simulink model "bb01_quick_start"  (Simulink 7.7)
settings: Solver=FixedStepDiscrete  StartTime=0.0  StopTime=inf  FixedStep=0.002  RelTol=1e-3
PostLoadFcn:
  | qc_set_target_type(getConfigSet(bdroot, 'QUARC Default Target Configuration'));
undefined symbols (not defined in the file): HIL, qc_get_step_size
libraries: quarc_library x5, simulink x2
settings Model: Creator=Rchan  LastModifiedBy=MLevis  SimulationMode=external  ExtModeTrigDuration=5000
settings SolverCC: PositivePriorityOrder=on
settings OptimizationCC: InitFltsAndDblsToZero=on
settings DebuggingCC: SaveWithParameterizedLinksMsg=none  MultiTaskDSMMsg=warning  MultiTaskCondExecSysMsg=none  StrictBusMsg=None
settings RTWCC: SystemTargetFile=quarc_win64.tlc  TemplateMakefile=quarc_default_tmf  Description=QUARC Win64 Target  ProcessScript=quarc_win64_make_rtw_hook
settings STFCustomTargetCC: TargetPreCompLibLocation=C:\PROGRA~3\QUARC\lib\2011a\win64\release  FunctionExecutionProfile=off  GeneratePreprocessorConditionals=Disable all  SystemTargetFile=quarc_win64.tlc
settings GRTTargetCC: TargetPreCompLibLocation=C:\PROGRA~3\QUARC\lib\2011a\win64\release  ParMdlRefBuildCompliant=off  CompOptLevelCompliant=off  MatFileLogging=off  ExtMode=on  ExtModeMexFile=quarc_comm

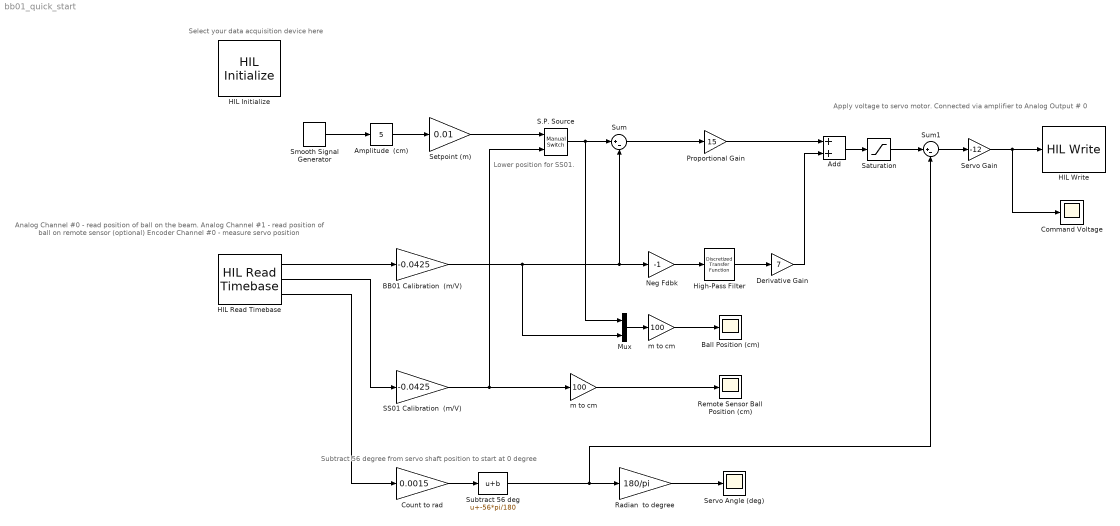
== system bb01_quick_start ==
  note: Select your data acquisition device here
  note: Lower position for SS01.
  note: Analog Channel #0 - read position of ball on the beam.
      | Analog Channel  #1 - read position of ball on remote sensor (optional)
      | Encoder Channel #0 - measure servo position
  note: Apply voltage to servo motor.
      | Connected via amplifier to Analog Output # 0
  note: Subtract 56 degree from servo shaft
      | position to start at 0 degree
  Add : Sum
  Amplitude  (cm) : simulink/Math Operations/Slider Gain  SystemSampleTime=-1  low=-10  gain=5  high=10
  BB01 Calibration  (m/V) : Gain  Gain=-0.0425  SaturateOnIntegerOverflow=on  OutDataTypeStr=Inherit: Same as input  ParamDataTypeStr=Inherit: Same as input
  Ball Position (cm) : Scope
      settings: YMin=-10  YMax=10  SaveName=ScopeData2
  Command Voltage : Scope
      settings: YMin=-10  YMax=10  SaveName=ScopeData3
  Count to rad : Gain  Gain=0.0015  SaturateOnIntegerOverflow=on  OutDataTypeStr=Inherit: Same as input  ParamDataTypeStr=Inherit: Same as input
  Derivative Gain : Gain  Gain=7
  HIL Initialize : quarc_library/Data Acquisition/Generic/Configuration/HIL Initialize  Priority=-99  object_name=HIL-1  board_type=q4  board_number=0  exclusive=off  active=off  hardware_clocks=[0:1]  clock_modes=[0 0]  initial_clock_frequencies=[]  set_clock_params_at_start=on  set_clock_params_at_switch_in=off  set_clock_frequencies_at_start=off  set_clock_frequencies_at_switch_in=off  analog_input_channels=[0:3]  analog_input_maximums=10  analog_input_minimums=-10  set_analog_input_params_at_start=off  set_analog_input_params_at_switch_in=off  analog_output_channels=[0:3]  analog_output_maximums=[10]  analog_output_minimums=[-10]  initial_analog_outputs=[0]  final_analog_outputs=[0]  watchdog_analog_outputs=0  set_analog_output_params_at_start=on  set_analog_output_params_at_switch_in=off  set_analog_outputs_at_start=on  set_analog_outputs_at_switch_in=off  set_analog_outputs_at_terminate=on  set_analog_outputs_at_switch_out=off  set_analog_outputs_on_watchdog=off  digital_input_channels=[]  digital_output_channels=[]  digital_output_configuration=[]  initial_digital_outputs=[1]  final_digital_outputs=[1]  watchdog_digital_outputs=[2]  set_digital_output_params_at_start=off  set_digital_output_params_at_switch_in=off  set_digital_outputs_at_start=on  set_digital_outputs_at_switch_in=off  set_digital_outputs_at_terminate=on  set_digital_outputs_at_switch_out=off  set_digital_outputs_on_watchdog=off  encoder_channels=[0:3]  quadrature=[4]  encoder_filter_frequency=(1/60e-9)/1  initial_encoder_counts=[0]  set_encoder_params_at_start=on  set_encoder_params_at_switch_in=off  set_encoder_counts_at_start=on  set_encoder_counts_at_switch_in=off  pwm_channels=[]  pwm_modes=[0]  pwm_frequency=(1/60e-9)/1024  pwm_configuration=[]  pwm_alignment=[]  pwm_polarity=[]  pwm_leading_deadband=[]  pwm_trailing_deadband=[]  initial_pwm_outputs=[0]  final_pwm_outputs=[0]  watchdog_pwm_outputs=[]  set_pwm_params_at_start=on  set_pwm_params_at_switch_in=off  set_pwm_outputs_at_start=on  set_pwm_outputs_at_switch_in=off  set_pwm_outputs_at_terminate=on  set_pwm_outputs_at_switch_out=off  set_pwm_outputs_on_watchdog=off  other_output_channels=[]  initial_other_outputs=[]  final_other_outputs=[]  watchdog_other_outputs=[]  set_other_outputs_at_start=off  set_other_outputs_at_switch_in=off  set_other_outputs_at_terminate=off  set_other_outputs_at_switch_out=off  set_other_outputs_on_watchdog=off
  HIL Read Timebase : quarc_library/Data Acquisition/Generic/Timebases/HIL Read Timebase  object_name=HIL-1  clock=0  analog_channels=0:1  encoder_channels=[0]  digital_channels=[]  other_channels=[]  samples_in_buffer=max(ceil(1/qc_get_step_size), 1)  active=on  vector_output=off  data_type_mode=Inherit via back propagation  encoder_data_type=double  digital_data_type=boolean
  HIL Write : quarc_library/Data Acquisition/Generic/Immediate I//O/HIL Write  object_name=HIL-1  analog_channels=0  pwm_channels=[]  digital_channels=[]  other_channels=[]  sample_time=-1  active=off  vector_input=off
  High-Pass Filter : quarc_library/Discrete/Discretized Transfer Function  SystemSampleTime=-1  num=[15 0]  den=[1 15]  method=tustin  Ts=qc_get_step_size
  Mux : Mux  Inputs=2
  Neg Fdbk : Gain  Gain=-1  SaturateOnIntegerOverflow=on  OutDataTypeStr=Inherit: Same as input  ParamDataTypeStr=Inherit: Same as input
  Proportional Gain : Gain  Gain=15
  "Radian  to degree " : Gain  Gain=180/pi  SaturateOnIntegerOverflow=on  OutDataTypeStr=Inherit: Same as input  ParamDataTypeStr=Inherit: Same as input
  Remote Sensor Ball Position (cm) : Scope
      settings: YMin=-10  YMax=10
  S.P. Source : simulink/Signal Routing/Manual Switch  SystemSampleTime=-1  sw=1  action=0  varsize=off
  SS01 Calibration  (m/V) : Gain  Gain=-0.0425  SaturateOnIntegerOverflow=on  OutDataTypeStr=Inherit: Same as input  ParamDataTypeStr=Inherit: Same as input
  Saturation : Saturate  UpperLimit=0.9774  LowerLimit=-0.9774
  Servo Angle (deg) : Scope
      settings: YMin=-60  YMax=60
  Servo Gain : Gain  Gain=-12
  Setpoint (m) : Gain  Gain=0.01
  Smooth Signal Generator : quarc_library/Sources/Signals/Smooth Signal Generator  signal_type=Square  source=Internal (dialog parameters)  amplitude=1  frequency=0.08  initial_phase=0  sample_time=qc_get_step_size  output_cos=off
  Subtract 56 deg : Bias  Bias=-56*pi/180
  Sum : Sum  Inputs=|+-
  Sum1 : Sum  Inputs=|+-
  m to cm : Gain  Gain=100  SaturateOnIntegerOverflow=on  OutDataTypeStr=Inherit: Same as input  ParamDataTypeStr=Inherit: Same as input
  "m to cm " : Gain  Gain=100  SaturateOnIntegerOverflow=on  OutDataTypeStr=Inherit: Same as input  ParamDataTypeStr=Inherit: Same as input
  wires:
  Smooth Signal Generator/1 -> Amplitude  (cm)/1
  Amplitude  (cm)/1 -> Setpoint (m)/1
  Sum/1 -> Proportional Gain/1
  Setpoint (m)/1 -> S.P. Source/1
  HIL Read Timebase/2 -> SS01 Calibration  (m/V)/1
  HIL Read Timebase/1 -> BB01 Calibration  (m/V)/1
  S.P. Source/1 -> Sum/1, Mux/1
  SS01 Calibration  (m/V)/1 -> S.P. Source/2, "m to cm "/1
  BB01 Calibration  (m/V)/1 -> Sum/2, Neg Fdbk/1, Mux/2
  HIL Read Timebase/3 -> Count to rad/1
  "Radian  to degree "/1 -> Servo Angle (deg)/1
  Neg Fdbk/1 -> High-Pass Filter/1
  High-Pass Filter/1 -> Derivative Gain/1
  Proportional Gain/1 -> Add/1
  Derivative Gain/1 -> Add/2
  Servo Gain/1 -> HIL Write/1, Command Voltage/1
  Add/1 -> Saturation/1
  Sum1/1 -> Servo Gain/1
  "m to cm "/1 -> Remote Sensor Ball Position (cm)/1
  m to cm/1 -> Ball Position (cm)/1
  Saturation/1 -> Sum1/1
  Count to rad/1 -> Subtract 56 deg/1
  Subtract 56 deg/1 -> "Radian  to degree "/1, Sum1/2
  Mux/1 -> m to cm/1
